simulink model "gpc_siso_2_sim"  (R2022a)
settings: Solver=VariableStepAuto  StartTime=0.0  StopTime=Tsim  RelTol=1e-3
undefined symbols (not defined in the file): a, A, Ab, b, Bb, D, F, Fb, H, Hb, K, Ko, Kr, Ts
libraries: cstblocks x1
settings Model: Creator=aaron  LastModifiedBy=aaron
settings SolverCC: AlgebraicLoopSolver=TrustRegion
settings DebuggingCC: UnconnectedInputMsg=warning  UnconnectedOutputMsg=warning  UnconnectedLineMsg=warning  SFMachineParentedDataDiag=warning

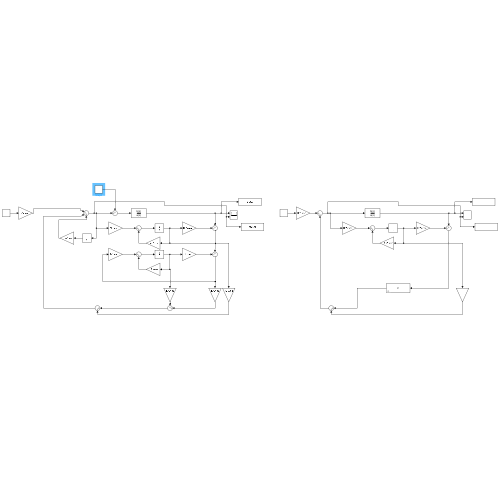
[thumbnail: Simulink's stored preview of the top-level diagram]
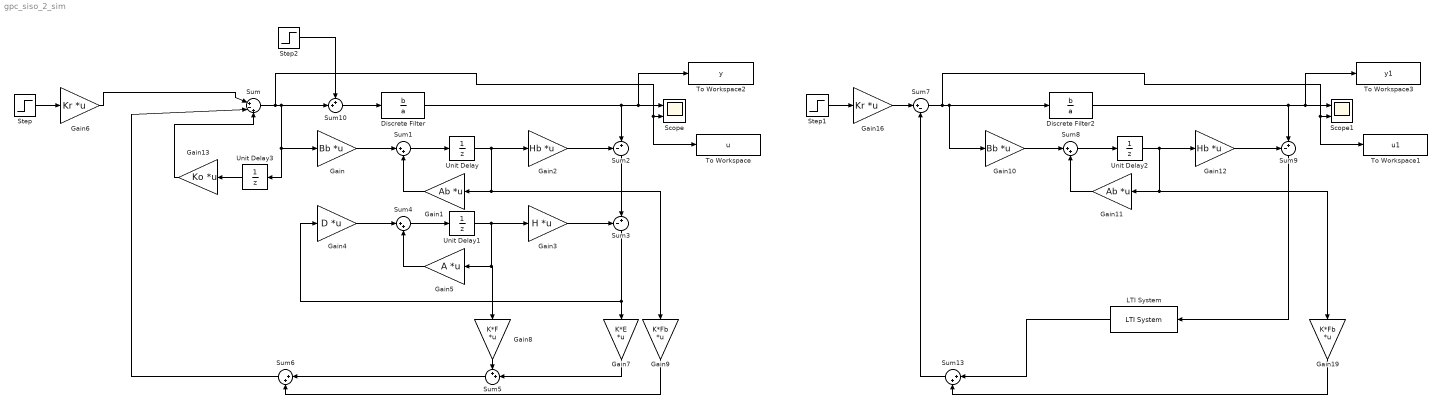
== system gpc_siso_2_sim ==
  Discrete Filter : DiscreteFilter  Numerator=b  Denominator=a
  Discrete Filter2 : DiscreteFilter  Numerator=b  Denominator=a
  Gain : Gain  Gain=Bb  Multiplication=Matrix(K*u) (u vector)
  Gain1 : Gain  Gain=Ab  Multiplication=Matrix(K*u) (u vector)
  Gain10 : Gain  Gain=Bb  Multiplication=Matrix(K*u) (u vector)
  Gain11 : Gain  Gain=Ab  Multiplication=Matrix(K*u) (u vector)
  Gain12 : Gain  Gain=Hb  Multiplication=Matrix(K*u) (u vector)
  Gain13 : Gain  Gain=Ko  Multiplication=Matrix(K*u) (u vector)
  Gain16 : Gain  Gain=Kr  Multiplication=Matrix(K*u) (u vector)
  Gain19 : Gain  Gain=K*Fb  Multiplication=Matrix(K*u) (u vector)
  Gain2 : Gain  Gain=Hb  Multiplication=Matrix(K*u) (u vector)
  Gain3 : Gain  Gain=H  Multiplication=Matrix(K*u) (u vector)
  Gain4 : Gain  Gain=D  Multiplication=Matrix(K*u) (u vector)
  Gain5 : Gain  Gain=A  Multiplication=Matrix(K*u) (u vector)
  Gain6 : Gain  Gain=Kr  Multiplication=Matrix(K*u) (u vector)
  Gain7 : Gain  Gain=K*E  Multiplication=Matrix(K*u) (u vector)
  Gain8 : Gain  Gain=K*F  Multiplication=Matrix(K*u) (u vector)
  Gain9 : Gain  Gain=K*Fb  Multiplication=Matrix(K*u) (u vector)
  LTI System : cstblocks/LTI System  sys=V  IC=[]
  Scope : Scope  NumInputPorts=2
  Scope1 : Scope  NumInputPorts=2
  Step : Step  Time=0  SampleTime=0
  Step1 : Step  Time=0  SampleTime=0
  Step2 : Step  Time=10  After=0.5  SampleTime=0
  Sum : Sum  Inputs=|+-+
  Sum{1,4,6,8,13} (5 alike) : Sum  Inputs=|++
  Sum10 : Sum  Inputs=++|
  Sum2 : Sum  Inputs=-+|
  Sum3 : Sum  Inputs=-+|
  Sum5 : Sum  Inputs=++|
  Sum7 : Sum  Inputs=|+-
  Sum9 : Sum  Inputs=-+|
  To Workspace : ToWorkspace  VariableName=u  SampleTime=Ts
  To Workspace1 : ToWorkspace  VariableName=u1  SampleTime=Ts
  To Workspace2 : ToWorkspace  VariableName=y  SampleTime=Ts
  To Workspace3 : ToWorkspace  VariableName=y1  SampleTime=Ts
  Unit Delay{,1..3} (4 alike) : UnitDelay  SampleTime=-1  HasFrameUpgradeWarning=on
  wires:
  Sum/1 -> To Workspace/1, Scope/2, Sum10/2, Gain/1, Unit Delay3/1
  Gain6/1 -> Sum/1
  Step/1 -> Gain6/1
  Gain/1 -> Sum1/1
  Sum1/1 -> Unit Delay/1
  Gain1/1 -> Sum1/2
  Unit Delay/1 -> Gain2/1, Gain9/1, Gain1/1
  Gain2/1 -> Sum2/1
  Discrete Filter/1 -> To Workspace2/1, Scope/1, Sum2/2
  Gain3/1 -> Sum3/1
  Sum2/1 -> Sum3/2
  Unit Delay1/1 -> Gain3/1, Gain5/1, Gain8/1
  Gain5/1 -> Sum4/2
  Sum4/1 -> Unit Delay1/1
  Gain4/1 -> Sum4/1
  Sum3/1 -> Gain7/1, Gain4/1
  Gain8/1 -> Sum5/1
  Gain7/1 -> Sum5/2
  Sum6/1 -> Sum/2
  Gain9/1 -> Sum6/2
  Sum5/1 -> Sum6/1
  Gain19/1 -> Sum13/2
  Sum13/1 -> Sum7/2
  Sum9/1 -> LTI System/1
  Discrete Filter2/1 -> Sum9/2, Scope1/1, To Workspace3/1
  Gain12/1 -> Sum9/1
  Unit Delay2/1 -> Gain11/1, Gain19/1, Gain12/1
  Gain11/1 -> Sum8/2
  Sum8/1 -> Unit Delay2/1
  Gain10/1 -> Sum8/1
  Step1/1 -> Gain16/1
  Gain16/1 -> Sum7/1
  Sum7/1 -> Discrete Filter2/1, Gain10/1, Scope1/2, To Workspace1/1
  LTI System/1 -> Sum13/1
  Sum10/1 -> Discrete Filter/1
  Step2/1 -> Sum10/1
  Gain13/1 -> Sum/3
  Unit Delay3/1 -> Gain13/1
